simulink model "orientation_control"  (R2024b)
settings: Solver=FixedStepAuto  StartTime=0.0  StopTime=t_end  FixedStep=dt  RelTol=1e-3
undefined symbols (not defined in the file or in its folder): kR, theta_init, theta_r
settings Model: Creator=yamauchi  LastModifiedBy=yamauchi

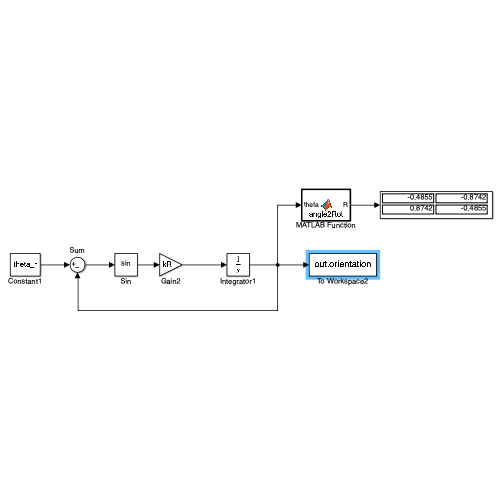
[thumbnail: Simulink's stored preview of the top-level diagram]
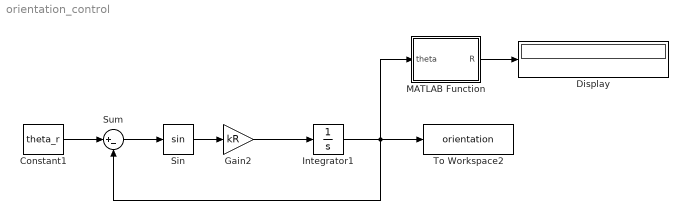
== system orientation_control ==
  Constant1 : Constant  Value=theta_r
  Display : Display
  Gain2 : Gain  Gain=kR
  Integrator1 : Integrator  InitialCondition=theta_init
  MATLAB Function : MATLAB Function  TreatAsAtomicUnit=on
  Sin : Trigonometry
  Sum : Sum  Inputs=|+-
  To Workspace2 : ToWorkspace  VariableName=orientation  SampleTime=-1
      settings: Save2DSignal=2-D array (concatenate along first dimension)
  wires:
  Sum/1 -> Sin/1
  Integrator1/1 -> MATLAB Function/1(theta), To Workspace2/1, Sum/2
  Constant1/1 -> Sum/1
  Gain2/1 -> Integrator1/1
  Sin/1 -> Gain2/1
  MATLAB Function/1(R) -> Display/1

== matlab function orientation_control/MATLAB Function ==
  data: theta input; R output
function R = angle2Rot(theta)

R = [cos(theta) -sin(theta); sin(theta) cos(theta)];
